simulink model "VTOL_sim"  (R2018a)
settings: Solver=ode45  StartTime=0.0  StopTime=100  RelTol=1e-3  EnableMultiTasking=on
InitFcn:
  | addpath ./..
  | VTOL_param
  | VTOLParamHW8
undefined symbols (not defined in the file or in its folder): P, VTOL_animation
settings Model: Creator=beard  LastModifiedBy=mclain
settings DataIOCC: LimitDataPoints=on  SaveFormat=Array  SignalLoggingSaveFormat=ModelDataLogs
settings OptimizationCC: ExpressionDepthLimit=2147483647  InitFltsAndDblsToZero=on  LifeSpan=inf
settings DebuggingCC: UnderspecifiedInitializationDetection=Classic  MergeDetectMultiDrivingBlocksExec=none  SolverPrmCheckMsg=warning  FcnCallInpInsideContextMsg=warning  StateNameClashWarn=warning  SFUnexpectedBacktrackingDiag=warning  SFNoUnconditionalDefaultTransitionDiag=warning  SFExecutionAtInitializationDiag=none
settings HardwareCC: ProdBitPerPointer=32  ProdBitPerSizeT=32  ProdBitPerPtrDiffT=32  ProdLargestAtomicFloat=None  ProdIntDivRoundTo=Undefined  ProdEndianess=Unspecified  ProdWordSize=32  ProdHWDeviceType=32-bit Generic
settings ModelReferenceCC: PropagateSignalLabelsOutOfModel=off
settings CodeAppCC: StateflowObjectComments=on
settings GRTTargetCC: TargetLangStandard=C89/C90 (ANSI)  GeneratePreprocessorConditionals=Disable all  CombineOutputUpdateFcns=off  GRTInterface=on
settings ConfigComp: CovMetricSettings=dw  CovHtmlReporting=on  CovSaveCumulativeToWorkspaceVar=on  CovSaveSingleToWorkspaceVar=on  CovExternalEMLEnable=off

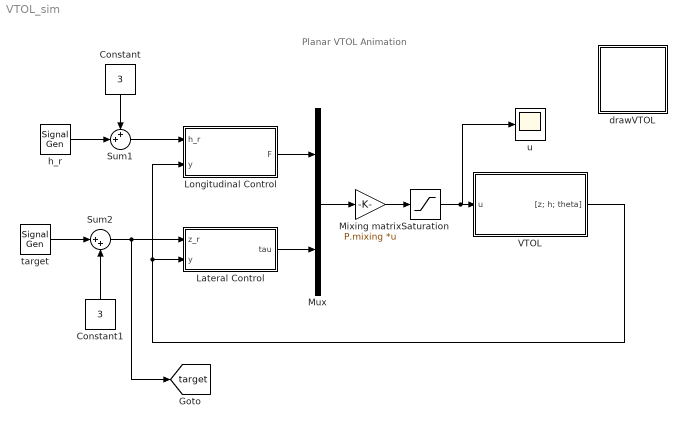
== system VTOL_sim ==
  note: Planar VTOL Animation
  Constant : Constant  Value=3
  Constant1 : Constant  Value=3
  Lateral Control : Subsystem
  Longitudinal Control : Subsystem
  Mixing matrix : Gain  Gain=P.mixing  Multiplication=Matrix(K*u)
  Mux : Mux  Inputs=2
  Saturation : Saturate  UpperLimit=P.fmax  LowerLimit=0
  Sum1 : Sum  Inputs=++|
  Sum2 : Sum  Inputs=|++
  VTOL : Subsystem
  drawVTOL : Subsystem
      mask Display: image(imread('tv.jpg'))
  h_r : SignalGenerator  WaveForm=square  Amplitude=2.5  Frequency=.03
  target : SignalGenerator  WaveForm=square  Amplitude=2.5  Frequency=.02
  u : Scope
  tag scope: target=global
  wires:
  VTOL/1("[z; h; theta]") -> Longitudinal Control/2(y), Lateral Control/2(y)
  Mux/1 -> Mixing matrix/1
  Mixing matrix/1 -> Saturation/1
  Longitudinal Control/1(F) -> Mux/1
  Lateral Control/1(tau) -> Mux/2
  Constant/1 -> Sum1/1
  Sum1/1 -> Longitudinal Control/1(h_r)
  h_r/1 -> Sum1/2
  target/1 -> Sum2/1
  Constant1/1 -> Sum2/2
  Saturation/1 -> u/1, VTOL/1(u)
  Sum2/1 -> [target], Lateral Control/1(z_r)

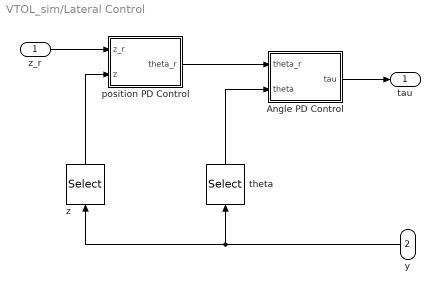
== system VTOL_sim/Lateral Control ==
  z_r : Inport
  y : Inport  Port=2
  "Angle PD Control " : Subsystem
  position PD Control : Subsystem
  theta : Selector  InputPortWidth=3  IndexOptions=Index vector (dialog)  Indices=[3]  OutputSizes=1
  z : Selector  InputPortWidth=3  IndexOptions=Index vector (dialog)  Indices=[1]  OutputSizes=1
  tau : Outport
  wires:
  y/1 -> z/1, theta/1
  position PD Control/1(theta_r) -> "Angle PD Control "/1(theta_r)
  theta/1 -> "Angle PD Control "/2(theta)
  z_r/1 -> position PD Control/1(z_r)
  z/1 -> position PD Control/2(z)
  "Angle PD Control "/1(tau) -> tau/1

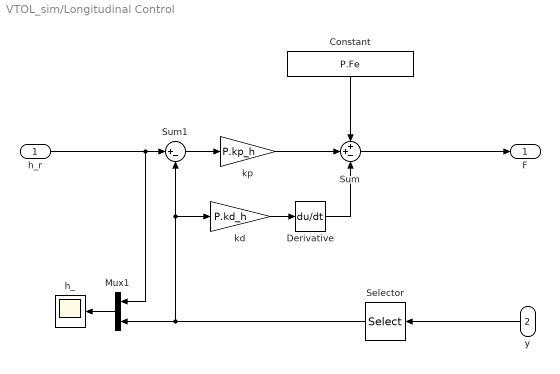
== system VTOL_sim/Longitudinal Control ==
  h_r : Inport
  y : Inport  Port=2
  Constant : Constant  Value=P.Fe
  Derivative : Derivative
  Mux1 : Mux  Inputs=2
  Selector : Selector  InputPortWidth=3  IndexOptions=Index vector (dialog)  Indices=[2]  OutputSizes=1
  Sum : Sum  Inputs=++-
  Sum1 : Sum  Inputs=|+-
  h_ : Scope
  kd : Gain  Gain=P.kd_h
  kp : Gain  Gain=P.kp_h
  F : Outport
  wires:
  Selector/1 -> kd/1, Sum1/2, Mux1/2
  Derivative/1 -> Sum/3
  Sum/1 -> F/1
  Mux1/1 -> h_/1
  kd/1 -> Derivative/1
  Constant/1 -> Sum/1
  h_r/1 -> Sum1/1, Mux1/1
  Sum1/1 -> kp/1
  y/1 -> Selector/1
  kp/1 -> Sum/2

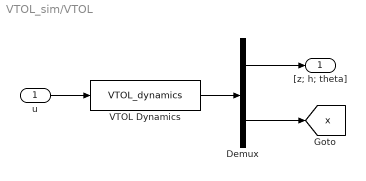
== system VTOL_sim/VTOL ==
  u : Inport
  Demux : Demux  Outputs=[3;6]
  VTOL Dynamics : S-Function  FunctionName=VTOL_dynamics  Parameters=P  SFunctionDeploymentMode=off  EnableBusSupport=off
  "[z; h; theta]" : Outport
  tag scope: x=global
  wires:
  u/1 -> VTOL Dynamics/1
  VTOL Dynamics/1 -> Demux/1
  Demux/1 -> "[z; h; theta]"/1
  Demux/2 -> [x]

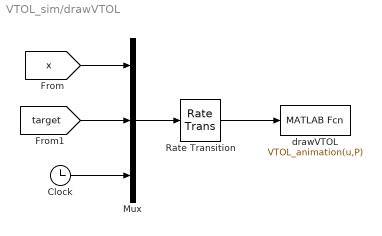
== system VTOL_sim/drawVTOL ==
  Clock : Clock
  Mux : Mux  Inputs=3
  Rate Transition : RateTransition  OutPortSampleTime=P.t_plot*10
  drawVTOL : MATLABFcn  MATLABFcn=VTOL_animation(u,P)  OutputDimensions=0
  wires:
  Mux/1 -> Rate Transition/1
  [x] -> Mux/1
  Clock/1 -> Mux/3
  Rate Transition/1 -> drawVTOL/1
  [target] -> Mux/2

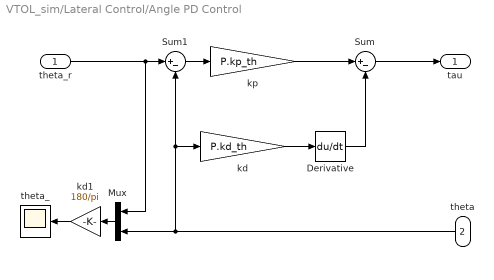
== system VTOL_sim/Lateral Control/Angle PD Control  ==
  theta_r : Inport
  theta : Inport  Port=2
  Derivative : Derivative
  Mux : Mux  Inputs=2
  Sum : Sum  Inputs=|+-
  Sum1 : Sum  Inputs=|+-
  kd : Gain  Gain=P.kd_th
  kd1 : Gain  Gain=180/pi
  kp : Gain  Gain=P.kp_th
  theta_ : Scope
  tau : Outport
  wires:
  theta_r/1 -> Sum1/1, Mux/1
  Sum/1 -> tau/1
  theta/1 -> kd/1, Sum1/2, Mux/2
  Sum1/1 -> kp/1
  kd1/1 -> theta_/1
  kp/1 -> Sum/1
  Mux/1 -> kd1/1
  kd/1 -> Derivative/1
  Derivative/1 -> Sum/2

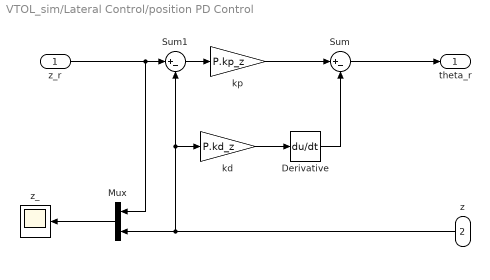
== system VTOL_sim/Lateral Control/position PD Control ==
  z_r : Inport
  z : Inport  Port=2
  Derivative : Derivative
  Mux : Mux  Inputs=2
  Sum : Sum  Inputs=|+-
  Sum1 : Sum  Inputs=|+-
  kd : Gain  Gain=P.kd_z
  kp : Gain  Gain=P.kp_z
  z_ : Scope
  theta_r : Outport
  wires:
  z_r/1 -> Sum1/1, Mux/1
  Sum/1 -> theta_r/1
  z/1 -> kd/1, Sum1/2, Mux/2
  Sum1/1 -> kp/1
  Mux/1 -> z_/1
  kp/1 -> Sum/1
  kd/1 -> Derivative/1
  Derivative/1 -> Sum/2
